simulink model "s1"  (R2023b)
settings: Solver=ode45  StartTime=1  StopTime=2  RelTol=1e-3
settings Model: Creator=t3  LastModifiedBy=t3

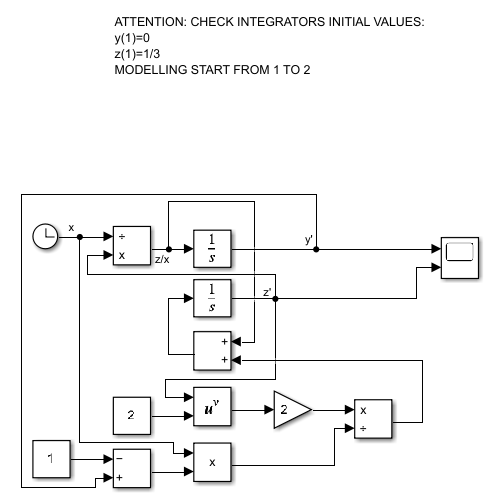
[thumbnail: Simulink's stored preview of the top-level diagram]
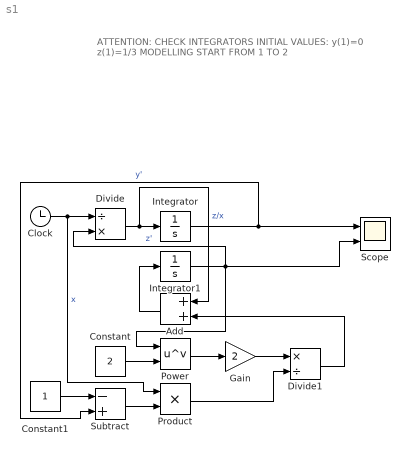
== system s1 ==
  note: ATTENTION: CHECK INTEGRATORS INITIAL VALUES:
      | y(1)=0
      | z(1)=1/3
      | MODELLING START FROM 1 TO 2
  Add : Sum
  Clock : Clock
  Constant : Constant  Value=2
  Constant1 : Constant
  Divide : Product  Inputs=/*
  Divide1 : Product  Inputs=*/
  Gain : Gain  Gain=2
  Integrator : Integrator
  Integrator1 : Integrator  InitialCondition=1/3
  Power : Math  Operator=pow
  Product : Product
  Scope : Scope  NumInputPorts=2
  Subtract : Sum  Inputs=-+
  wires:
  Clock/1 -> Product/1, Divide/1  "x"
  Divide/1 -> Add/1, Integrator/1  "z/x"
  Integrator/1 -> Subtract/2, Scope/1  "y'"
  Integrator1/1 -> Power/1, Divide/2, Scope/2  "z'"
  Add/1 -> Integrator1/1
  Constant/1 -> Power/2
  Power/1 -> Gain/1
  Gain/1 -> Divide1/1
  Product/1 -> Divide1/2
  Subtract/1 -> Product/2
  Constant1/1 -> Subtract/1
  Divide1/1 -> Add/2
